simulink model "RTInductionMotorJan27"  (R2019a)
settings: Solver=VariableStepAuto  StartTime=0.0  StopTime=1  RelTol=1e-3
model workspace (MAT data in the model file):
  Fe = 60
  Poles = 2
values from neighbouring files (symbols this model uses):
  Lm = 0.1485    [Setup.m]
  Lr = 0.009061    [Setup.m]
  Ls = 0.003883    [Setup.m]
  Rr = 1.06    [Setup.m]
  Rs = 1    [Setup.m]
libraries: powerlib_meascontrol x1
settings Model: Creator=adam_  LastModifiedBy=adam_

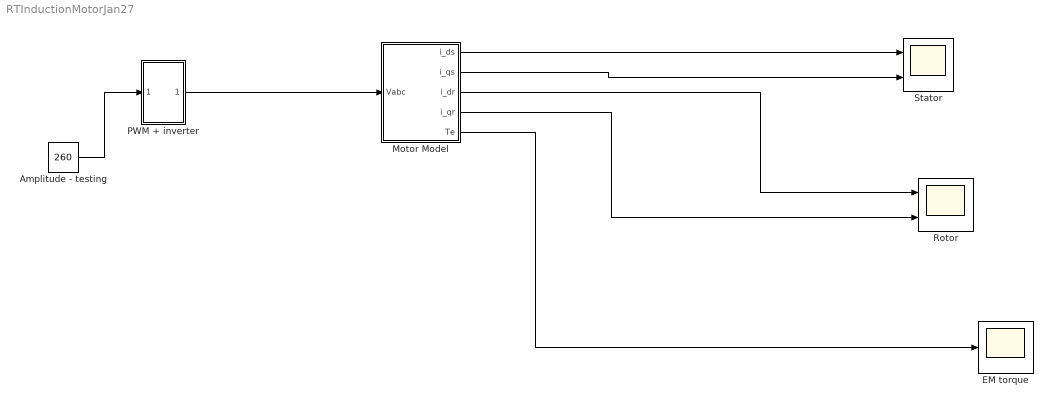
== system RTInductionMotorJan27 ==
  Amplitude - testing : Constant  Value=260
  EM torque : Scope
  Motor Model : Subsystem
  PWM + inverter : Subsystem
  Rotor : Scope  NumInputPorts=2
  Stator : Scope  NumInputPorts=2
  wires:
  PWM + inverter/1(Vabc) -> Motor Model/1(Vabc)
  Motor Model/1(i_ds) -> Stator/1
  Motor Model/2(i_qs) -> Stator/2
  Motor Model/3(i_dr) -> Rotor/1
  Motor Model/4(i_qr) -> Rotor/2
  Motor Model/5(Te) -> EM torque/1
  Amplitude - testing/1 -> PWM + inverter/1(Amplitude)

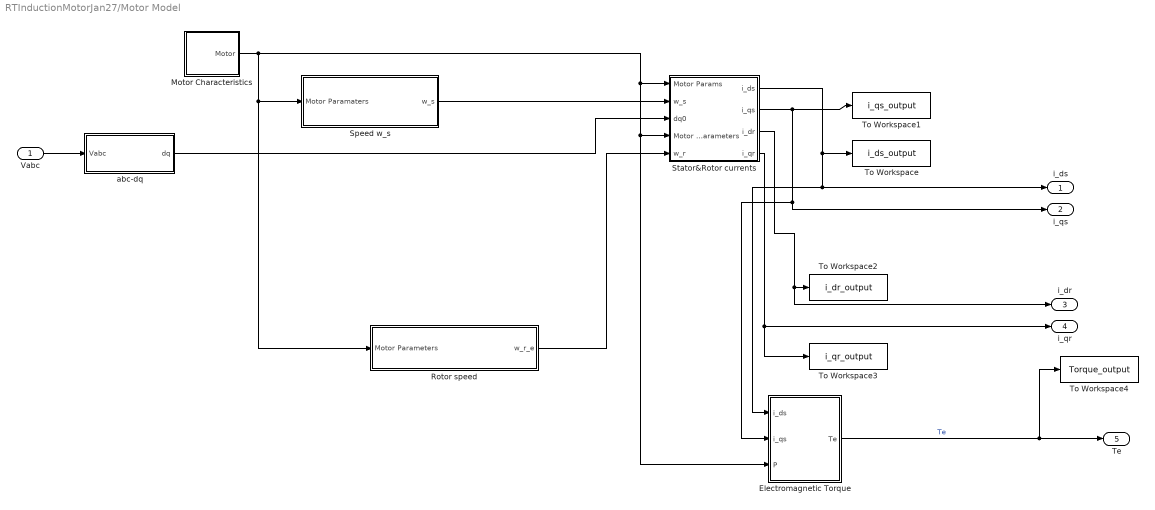
== system RTInductionMotorJan27/Motor Model ==
  Vabc : Inport
  Electromagnetic Torque : Subsystem
  Motor Characteristics : Subsystem
  Rotor speed : Subsystem
  Speed w_s : Subsystem
  Stator&Rotor currents : Subsystem
  To Workspace : ToWorkspace  VariableName=i_ds_output  SaveFormat=Timeseries  SampleTime=-1
  To Workspace1 : ToWorkspace  VariableName=i_qs_output  SaveFormat=Timeseries  SampleTime=-1
  To Workspace2 : ToWorkspace  VariableName=i_dr_output  SaveFormat=Timeseries  SampleTime=-1
  To Workspace3 : ToWorkspace  VariableName=i_qr_output  SaveFormat=Timeseries  SampleTime=-1
  To Workspace4 : ToWorkspace  VariableName=Torque_output  SaveFormat=Timeseries  SampleTime=-1
  abc-dq : Subsystem
  i_ds : Outport
  i_qs : Outport  Port=2
  i_dr : Outport  Port=3
  i_qr : Outport  Port=4
  Te : Outport  Port=5
  wires:
  Vabc/1 -> abc-dq/1(Vabc)
  Rotor speed/1(w_r_e) -> Stator&Rotor currents/5(w_r)
  abc-dq/1(dq) -> Stator&Rotor currents/3(dq0)
  Speed w_s/1(w_s) -> Stator&Rotor currents/2(w_s)
  Stator&Rotor currents/1(i_ds) -> i_ds/1, Electromagnetic Torque/1(i_ds), To Workspace/1
  Motor Characteristics/1(Motor) -> Rotor speed/1(Motor Parameters), Speed w_s/1(Motor Paramaters), Electromagnetic Torque/3(P), Stator&Rotor currents/4(Motor Parameters), Stator&Rotor currents/1(Motor Params)
  Stator&Rotor currents/2(i_qs) -> i_qs/1, Electromagnetic Torque/2(i_qs), To Workspace1/1
  Stator&Rotor currents/4(i_qr) -> i_qr/1, To Workspace3/1
  Stator&Rotor currents/3(i_dr) -> i_dr/1, To Workspace2/1
  Electromagnetic Torque/1(Te) -> Te/1, To Workspace4/1  "Te"

== system RTInductionMotorJan27/PWM + inverter ==
  Amplitude : Inport
  Mux : Mux  Inputs=3
  Product : Product
  Product1 : Product
  Product2 : Product
  Scope : Scope
  Sine Wave : Sin  Frequency=2*pi*60  SampleTime=0
  Sine Wave1 : Sin  Frequency=2*pi*60  Phase=2*pi/3  SampleTime=0
  Sine Wave2 : Sin  Frequency=2*pi*60  Phase=4*pi/3  SampleTime=0
  Three-phase PWM : Subsystem
  Vdc : Constant  Value=360
  inverter : Subsystem
  Vabc : Outport
  wires:
  Mux/1 -> Three-phase PWM/1(Signals)
  Three-phase PWM/1(Pulses) -> inverter/2(Pulses)
  inverter/1(Vabc) -> Vabc/1, Scope/1
  Vdc/1 -> inverter/1(Vdc)
  Sine Wave/1 -> Product/2
  Amplitude/1 -> Product2/1, Product1/1, Product/1
  Product/1 -> Mux/1
  Product2/1 -> Mux/3
  Product1/1 -> Mux/2
  Sine Wave1/1 -> Product1/2
  Sine Wave2/1 -> Product2/2

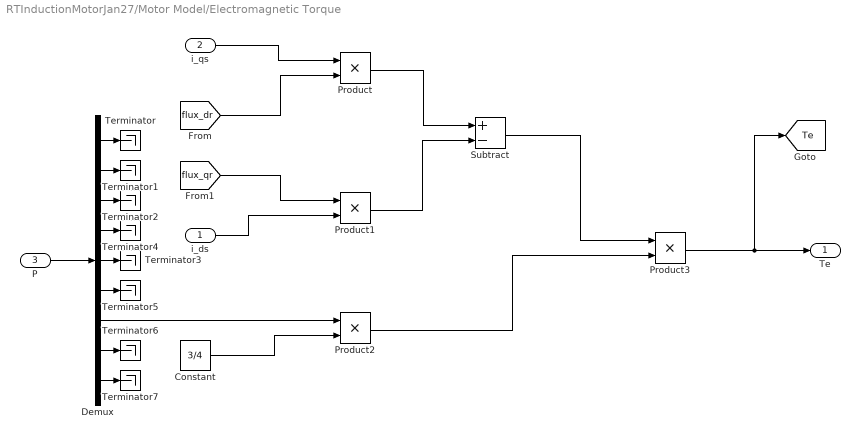
== system RTInductionMotorJan27/Motor Model/Electromagnetic Torque ==
  i_ds : Inport
  i_qs : Inport  Port=2
  P : Inport  Port=3
  Constant : Constant  Value=3/4
  Demux : Demux  Outputs=9
  Product{,1..3} (4 alike) : Product
  Subtract : Sum  Inputs=+-
  Terminator{,1..7} (8 alike) : Terminator
  Te : Outport  VectorParamsAs1DForOutWhenUnconnected=off
  tag scope: Te=global
  wires:
  Product3/1 -> Te/1, [Te]
  Subtract/1 -> Product3/1
  Product2/1 -> Product3/2
  Constant/1 -> Product2/2
  Product1/1 -> Subtract/2
  Product/1 -> Subtract/1
  i_ds/1 -> Product1/2
  [flux_qr] -> Product1/1
  [flux_dr] -> Product/2
  i_qs/1 -> Product/1
  P/1 -> Demux/1
  Demux/7 -> Product2/1
  Demux/1 -> Terminator/1
  Demux/2 -> Terminator1/1
  Demux/3 -> Terminator2/1
  Demux/5 -> Terminator3/1
  Demux/4 -> Terminator4/1
  Demux/6 -> Terminator5/1
  Demux/8 -> Terminator6/1
  Demux/9 -> Terminator7/1

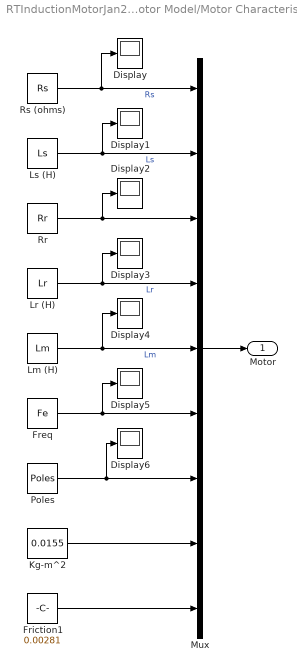
== system RTInductionMotorJan27/Motor Model/Motor Characteristics ==
  Display{,1..6} (7 alike) : Display
  Freq : Constant  Value=Fe
  Friction1 : Constant  Value=0.00281
  Kg-m^2 : Constant  Value=0.0155
  Lm (H) : Constant  Value=Lm
  Lr (H) : Constant  Value=Lr
  Ls (H) : Constant  Value=Ls
  Mux : Mux  Inputs=9
  Poles : Constant  Value=Poles
  Rr : Constant  Value=Rr
  Rs (ohms) : Constant  Value=Rs
  Motor : Outport
  wires:
  Rs (ohms)/1 -> Display/1, Mux/1  "Rs"
  Ls (H)/1 -> Display1/1, Mux/2  "Ls"
  Mux/1 -> Motor/1
  Rr/1 -> Display2/1, Mux/3
  Lr (H)/1 -> Display3/1, Mux/4  "Lr"
  Lm (H)/1 -> Display4/1, Mux/5  "Lm"
  Freq/1 -> Display5/1, Mux/6
  Poles/1 -> Display6/1, Mux/7
  Kg-m^2/1 -> Mux/8
  Friction1/1 -> Mux/9

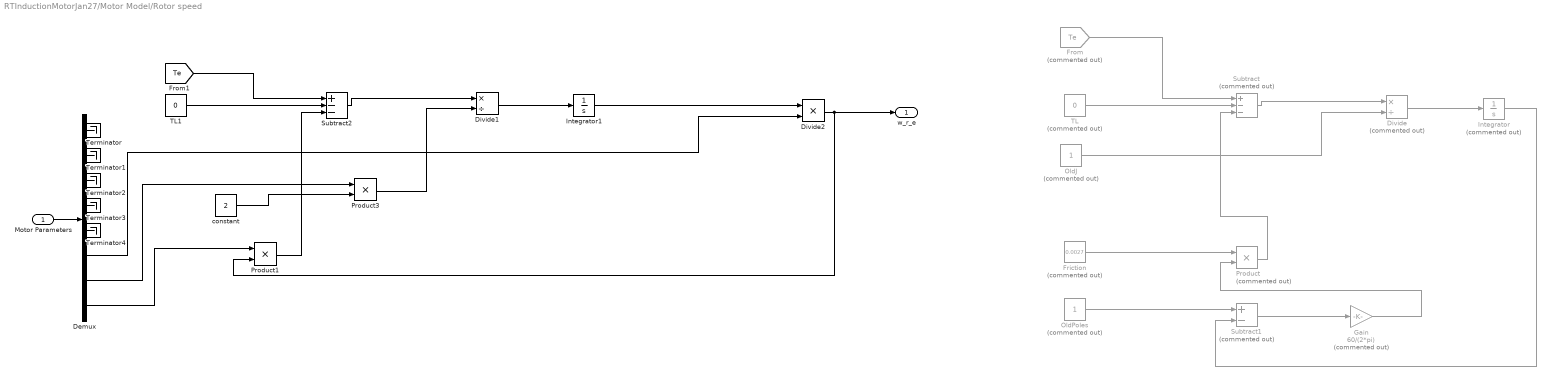
== system RTInductionMotorJan27/Motor Model/Rotor speed ==
  Motor Parameters : Inport
  Demux : Demux  Outputs=8
  Divide : Product  Commented=on  Inputs=*/
  Divide1 : Product  Inputs=*/
  Divide2 : Product  Inputs=**
  Friction : Constant  Commented=on  Value=0.0027
  From : From  Commented=on  GotoTag=Te  TagVisibility=global
  Gain : Gain  Commented=on  Gain=60/(2*pi)
  Integrator : Integrator  Commented=on
  Integrator1 : Integrator
  OldJ : Constant  Commented=on
  OldPoles : Constant  Commented=on
  Product : Product  Commented=on
  Product1 : Product
  Product3 : Product
  Subtract : Sum  Commented=on  Inputs=+--
  Subtract1 : Sum  Commented=on  Inputs=+-
  Subtract2 : Sum  Inputs=+--
  TL : Constant  Commented=on  Value=0
  TL1 : Constant  Value=0
  Terminator{,1..4} (5 alike) : Terminator
  constant : Constant  Value=2
  w_r_e : Outport  VectorParamsAs1DForOutWhenUnconnected=off
  wires:
  From/1 -> Subtract/1
  TL/1 -> Subtract/2
  Subtract/1 -> Divide/1
  Divide/1 -> Integrator/1
  Integrator/1 -> Subtract1/2
  Subtract1/1 -> Gain/1
  Gain/1 -> Product/2
  Friction/1 -> Product/1
  Product/1 -> Subtract/3
  [Te] -> Subtract2/1
  Subtract2/1 -> Divide1/1
  Divide1/1 -> Integrator1/1
  TL1/1 -> Subtract2/2
  Product1/1 -> Subtract2/3
  constant/1 -> Product3/2
  Product3/1 -> Divide1/2
  Integrator1/1 -> Divide2/1
  Demux/6 -> Divide2/2
  Divide2/1 -> Product1/2, w_r_e/1
  Motor Parameters/1 -> Demux/1
  Demux/7 -> Product3/1
  Demux/8 -> Product1/1
  OldJ/1 -> Divide/2
  OldPoles/1 -> Subtract1/1

== system RTInductionMotorJan27/Motor Model/Speed w_s ==
  Motor Paramaters : Inport
  Demux : Demux  Outputs=9
  Divide2 : Product  Inputs=**/
  Terminator{,1..5,7} (7 alike) : Terminator
  constant1 : Constant  Value=120
  rpm to rad/s : Gain  Gain=2*pi/60
  w_s : Outport  VectorParamsAs1DForOutWhenUnconnected=off
  wires:
  constant1/1 -> Divide2/1
  Divide2/1 -> rpm to rad/s/1  "n_s"
  rpm to rad/s/1 -> w_s/1
  Motor Paramaters/1 -> Demux/1
  Demux/6 -> Divide2/2
  Demux/7 -> Divide2/3
  Demux/8 -> Terminator5/1

== system RTInductionMotorJan27/Motor Model/Stator&Rotor currents ==
  Motor Params : Inport
  w_s : Inport  Port=2
  dq0 : Inport  Port=3
  Motor Parameters : Inport  Port=4
  w_r : Inport  Port=5
  Rotor current : Subsystem
  Stator current : Subsystem
  i_ds : Outport
  i_qs : Outport  Port=2
  i_dr : Outport  Port=3
  i_qr : Outport  Port=4
  wires:
  w_s/1 -> Rotor current/2(w_s), Stator current/2(w_s)
  dq0/1 -> Stator current/3(dq0)
  w_r/1 -> Rotor current/3(w_r)
  Stator current/2(i_qs) -> i_qs/1
  Rotor current/1(i_dr) -> i_dr/1
  Motor Parameters/1 -> Rotor current/1(Motor Parameters)
  Motor Params/1 -> Stator current/1(Motor Params)
  Stator current/1(i_ds) -> i_ds/1
  Rotor current/2(i_qr) -> i_qr/1

== system RTInductionMotorJan27/Motor Model/abc-dq ==
  Vabc : Inport
  Add : Sum
  Constant : Constant  Value=2*pi*60
  Constant1 : Constant  Value=-pi/3
  Integrator : Integrator
  Mux3 : Mux  Inputs=2
  Mux4 : Mux  Inputs=2
  Scope2 : Scope
  Scope3 : Scope
  Vd : Fcn  Expr=sqrt(2/3)*(u(1)*cos(u(4))+u(2)*cos(u(4)-2*pi/3)+u(3)*cos(u(4)+2*pi/3))
  Vq : Fcn  Expr=-sqrt(2/3)*(u(1)*sin(u(4))+u(2)*sin(u(4)-2*pi/3)+u(3)*sin(u(4)+2*pi/3))
  dq : Outport  VectorParamsAs1DForOutWhenUnconnected=off
  wires:
  Vabc/1 -> Mux3/1
  Mux3/1 -> Vd/1, Vq/1, Scope2/1
  Constant/1 -> Integrator/1
  Integrator/1 -> Add/1  "w_t"
  Constant1/1 -> Add/2
  Vd/1 -> Mux4/1
  Vq/1 -> Mux4/2
  Mux4/1 -> dq/1, Scope3/1
  Add/1 -> Mux3/2

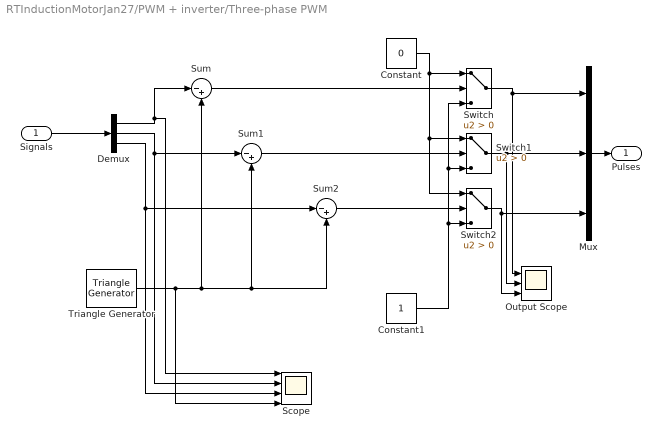
== system RTInductionMotorJan27/PWM + inverter/Three-phase PWM ==
  Signals : Inport
  Constant : Constant  Value=0
  Constant1 : Constant
  Demux : Demux  Outputs=3
  Mux : Mux  Inputs=3
  Output Scope : Scope  NumInputPorts=3
  Scope : Scope  NumInputPorts=4
  Sum : Sum  Inputs=|-+
  Sum1 : Sum  Inputs=|-+
  Sum2 : Sum  Inputs=|-+
  Switch : Switch  Criteria=u2 > Threshold
  Switch1 : Switch  Criteria=u2 > Threshold
  Switch2 : Switch  Criteria=u2 > Threshold
  Triangle Generator : powerlib_meascontrol/Pulse & Signal Generators/Triangle Generator  Freq=fs  Phase=90  Ts=1e-6
  Pulses : Outport
  wires:
  Sum/1 -> Switch/2
  Triangle Generator/1 -> Scope/4, Sum2/2, Sum1/2, Sum/2
  Constant/1 -> Switch2/1, Switch1/1, Switch/1
  Switch1/1 -> Output Scope/2, Mux/2
  Demux/2 -> Scope/2, Sum1/1
  Switch2/1 -> Output Scope/3, Mux/3
  Constant1/1 -> Switch1/3, Switch/3, Switch2/3
  Switch/1 -> Output Scope/1, Mux/1
  Demux/3 -> Scope/3, Sum2/1
  Sum1/1 -> Switch1/2
  Sum2/1 -> Switch2/2
  Mux/1 -> Pulses/1
  Signals/1 -> Demux/1
  Demux/1 -> Scope/1, Sum/1

== system RTInductionMotorJan27/PWM + inverter/inverter ==
  Vdc : Inport
  Pulses : Inport  Port=2
  Mux : Mux  Inputs=2
  Mux1 : Mux  Inputs=3
  Scope : Scope  NumInputPorts=3
  vaN : Fcn  Expr=u(1)*((2*u(2))-u(3)-u(4))/3
  vbN : Fcn  Expr=u(1)*((2*u(3))-u(2)-u(4))/3
  vcN : Fcn  Expr=u(1)*((2*u(4))-u(3)-u(2))/3
  Vabc : Outport
  wires:
  Vdc/1 -> Mux/1
  Pulses/1 -> Mux/2
  Mux/1 -> vcN/1, vbN/1, vaN/1
  Mux1/1 -> Vabc/1
  vaN/1 -> Scope/1, Mux1/1
  vbN/1 -> Scope/2, Mux1/2
  vcN/1 -> Mux1/3, Scope/3

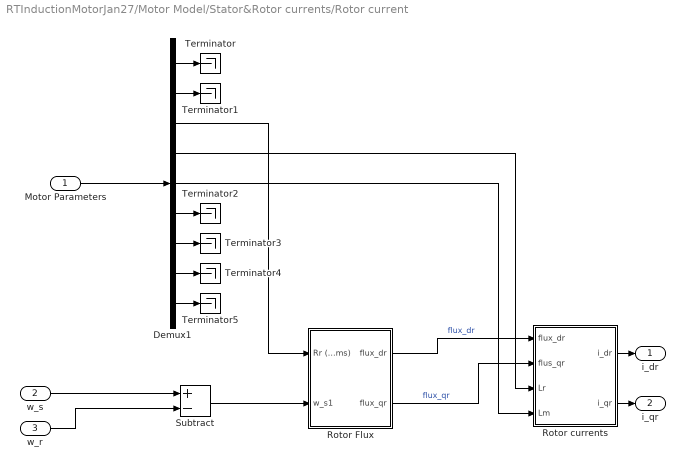
== system RTInductionMotorJan27/Motor Model/Stator&Rotor currents/Rotor current ==
  Motor Parameters : Inport
  w_s : Inport  Port=2
  w_r : Inport  Port=3
  Demux1 : Demux  Outputs=9
  Rotor Flux : Subsystem
  Rotor currents : Subsystem
  Subtract : Sum  Inputs=+-
  Terminator{,1..5} (6 alike) : Terminator
  i_dr : Outport  VectorParamsAs1DForOutWhenUnconnected=off
  i_qr : Outport  Port=2  VectorParamsAs1DForOutWhenUnconnected=off
  wires:
  Subtract/1 -> Rotor Flux/2(w_s1)
  w_r/1 -> Subtract/2
  Rotor currents/2(i_qr) -> i_qr/1
  Rotor currents/1(i_dr) -> i_dr/1
  Rotor Flux/1(flux_dr) -> Rotor currents/1(flux_dr)  "flux_dr"
  Rotor Flux/2(flux_qr) -> Rotor currents/2(flus_qr)  "flux_qr"
  w_s/1 -> Subtract/1
  Motor Parameters/1 -> Demux1/1
  Demux1/3 -> Rotor Flux/1(Rr (Ohms))
  Demux1/4 -> Rotor currents/3(Lr)
  Demux1/5 -> Rotor currents/4(Lm)
  Demux1/1 -> Terminator/1
  Demux1/2 -> Terminator1/1
  Demux1/6 -> Terminator2/1
  Demux1/7 -> Terminator3/1
  Demux1/8 -> Terminator4/1
  Demux1/9 -> Terminator5/1

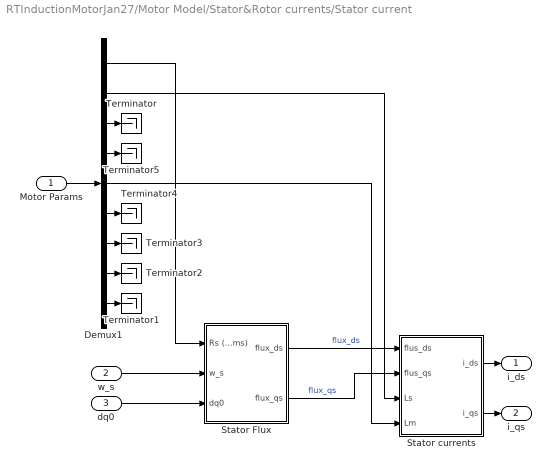
== system RTInductionMotorJan27/Motor Model/Stator&Rotor currents/Stator current ==
  Motor Params : Inport
  w_s : Inport  Port=2
  dq0 : Inport  Port=3
  Demux1 : Demux  Outputs=9
  Stator Flux : Subsystem
  Stator currents : Subsystem
  Terminator{,1..5} (6 alike) : Terminator
  i_ds : Outport  VectorParamsAs1DForOutWhenUnconnected=off
  i_qs : Outport  Port=2  VectorParamsAs1DForOutWhenUnconnected=off
  wires:
  dq0/1 -> Stator Flux/3(dq0)
  Stator currents/2(i_qs) -> i_qs/1
  w_s/1 -> Stator Flux/2(w_s)
  Stator currents/1(i_ds) -> i_ds/1
  Stator Flux/1(flux_ds) -> Stator currents/1(flus_ds)  "flux_ds"
  Stator Flux/2(flux_qs) -> Stator currents/2(flus_qs)  "flux_qs"
  Motor Params/1 -> Demux1/1
  Demux1/1 -> Stator Flux/1(Rs (Ohms))
  Demux1/2 -> Stator currents/3(Ls)
  Demux1/5 -> Stator currents/4(Lm)
  Demux1/3 -> Terminator/1
  Demux1/4 -> Terminator5/1
  Demux1/6 -> Terminator4/1
  Demux1/7 -> Terminator3/1
  Demux1/8 -> Terminator2/1
  Demux1/9 -> Terminator1/1

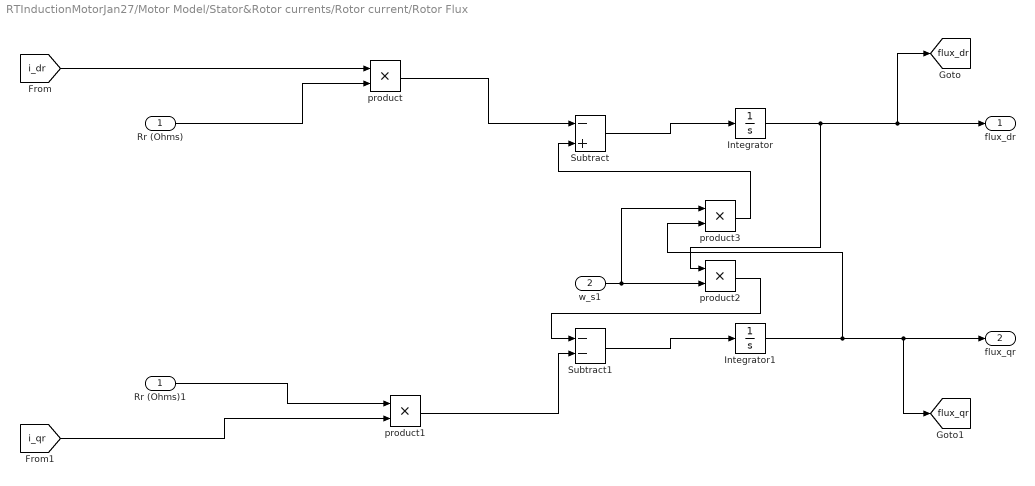
== system RTInductionMotorJan27/Motor Model/Stator&Rotor currents/Rotor current/Rotor Flux ==
  Rr (Ohms) : Inport
  w_s1 : Inport  Port=2
  Integrator : Integrator
  Integrator1 : Integrator
  Rr (Ohms)1 : InportShadow
  Subtract : Sum  Inputs=-+
  Subtract1 : Sum  Inputs=--
  product{,1..3} (4 alike) : Product  Inputs=**
  flux_dr : Outport  VectorParamsAs1DForOutWhenUnconnected=off
  flux_qr : Outport  Port=2  VectorParamsAs1DForOutWhenUnconnected=off
  tag scope: flux_dr=global, flux_qr=global
  wires:
  [i_qr] -> product1/2
  product2/1 -> Subtract1/1
  product3/1 -> Subtract/2
  w_s1/1 -> product2/2, product3/1
  Rr (Ohms)1/1 -> product1/1
  Integrator1/1 -> flux_qr/1, [flux_qr], product3/2
  [i_dr] -> product/1
  product1/1 -> Subtract1/2
  Subtract1/1 -> Integrator1/1
  Integrator/1 -> flux_dr/1, [flux_dr], product2/1
  Subtract/1 -> Integrator/1
  product/1 -> Subtract/1
  Rr (Ohms)/1 -> product/2

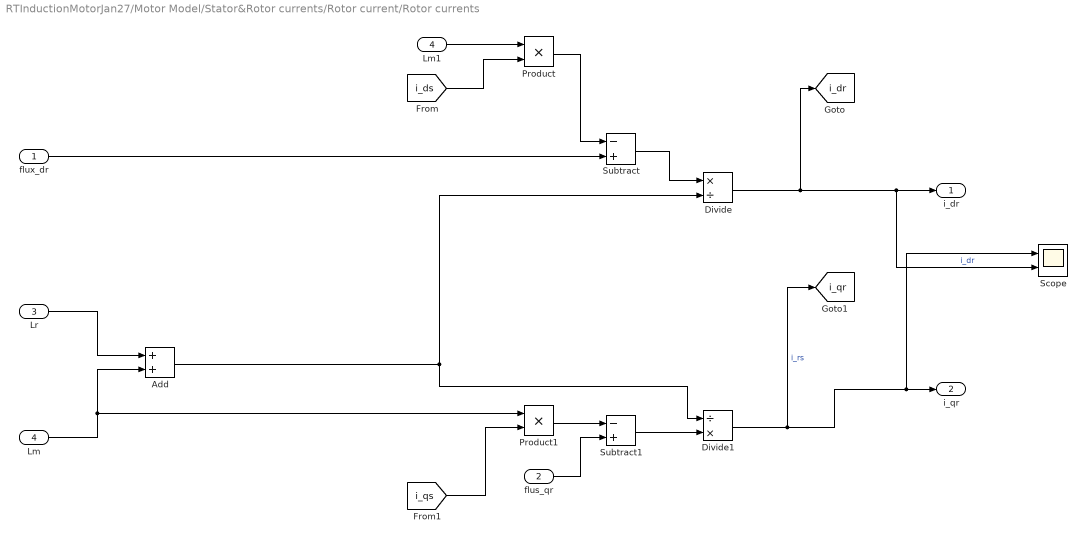
== system RTInductionMotorJan27/Motor Model/Stator&Rotor currents/Rotor current/Rotor currents ==
  flux_dr : Inport
  flus_qr : Inport  Port=2
  Lr : Inport  Port=3
  Lm : Inport  Port=4
  Add : Sum
  Divide : Product  Inputs=*/
  Divide1 : Product  Inputs=/*
  Lm1 : InportShadow  Port=4
  Product : Product
  Product1 : Product
  Scope : Scope  NumInputPorts=2
  Subtract : Sum  Inputs=-+
  Subtract1 : Sum  Inputs=-+
  i_dr : Outport  VectorParamsAs1DForOutWhenUnconnected=off
  i_qr : Outport  Port=2  VectorParamsAs1DForOutWhenUnconnected=off
  tag scope: i_dr=global, i_qr=global
  wires:
  Divide1/1 -> i_qr/1, Scope/1, [i_qr]  "i_rs"
  Subtract1/1 -> Divide1/2
  flus_qr/1 -> Subtract1/2
  Product1/1 -> Subtract1/1
  [i_qs] -> Product1/2
  Divide/1 -> i_dr/1, Scope/2, [i_dr]  "i_dr"
  Add/1 -> Divide/2, Divide1/1
  Subtract/1 -> Divide/1
  Lm/1 -> Add/2, Product1/1
  Lr/1 -> Add/1
  Product/1 -> Subtract/1
  flux_dr/1 -> Subtract/2
  [i_ds] -> Product/2
  Lm1/1 -> Product/1

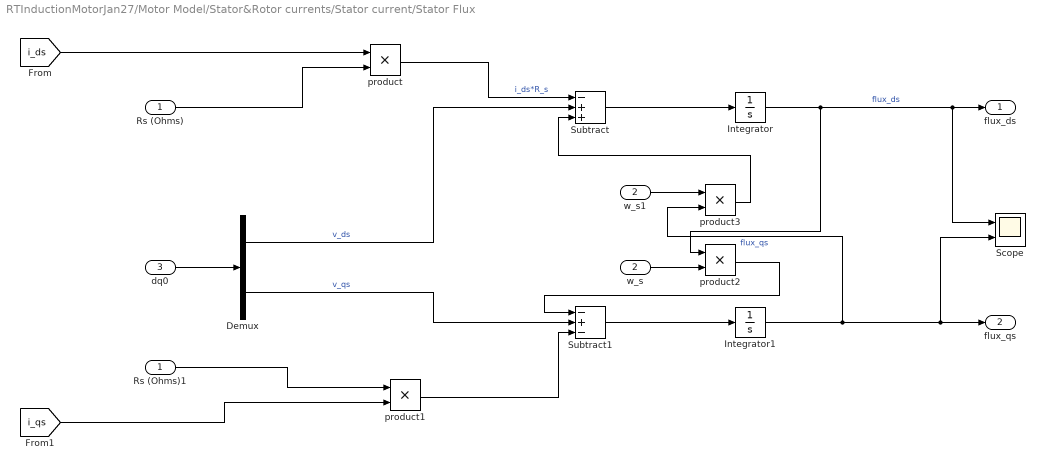
== system RTInductionMotorJan27/Motor Model/Stator&Rotor currents/Stator current/Stator Flux ==
  Rs (Ohms) : Inport
  w_s : Inport  Port=2
  dq0 : Inport  Port=3
  Demux : Demux  Outputs=2
  Integrator : Integrator
  Integrator1 : Integrator
  Rs (Ohms)1 : InportShadow
  Scope : Scope  NumInputPorts=2
  Subtract : Sum  Inputs=-++
  Subtract1 : Sum  Inputs=-+-
  product{,1..3} (4 alike) : Product  Inputs=**
  w_s1 : InportShadow  Port=2
  flux_ds : Outport  VectorParamsAs1DForOutWhenUnconnected=off
  flux_qs : Outport  Port=2  VectorParamsAs1DForOutWhenUnconnected=off
  wires:
  Demux/2 -> Subtract1/2  "v_qs"
  Demux/1 -> Subtract/2  "v_ds"
  [i_qs] -> product1/2
  product2/1 -> Subtract1/1
  w_s/1 -> product2/2
  product3/1 -> Subtract/3
  w_s1/1 -> product3/1
  Rs (Ohms)1/1 -> product1/1
  Integrator1/1 -> flux_qs/1, Scope/2, product3/2  "flux_qs"
  [i_ds] -> product/1
  product1/1 -> Subtract1/3
  Subtract1/1 -> Integrator1/1
  Integrator/1 -> flux_ds/1, Scope/1, product2/1  "flux_ds"
  Subtract/1 -> Integrator/1
  product/1 -> Subtract/1  "i_ds*R_s"
  Rs (Ohms)/1 -> product/2
  dq0/1 -> Demux/1

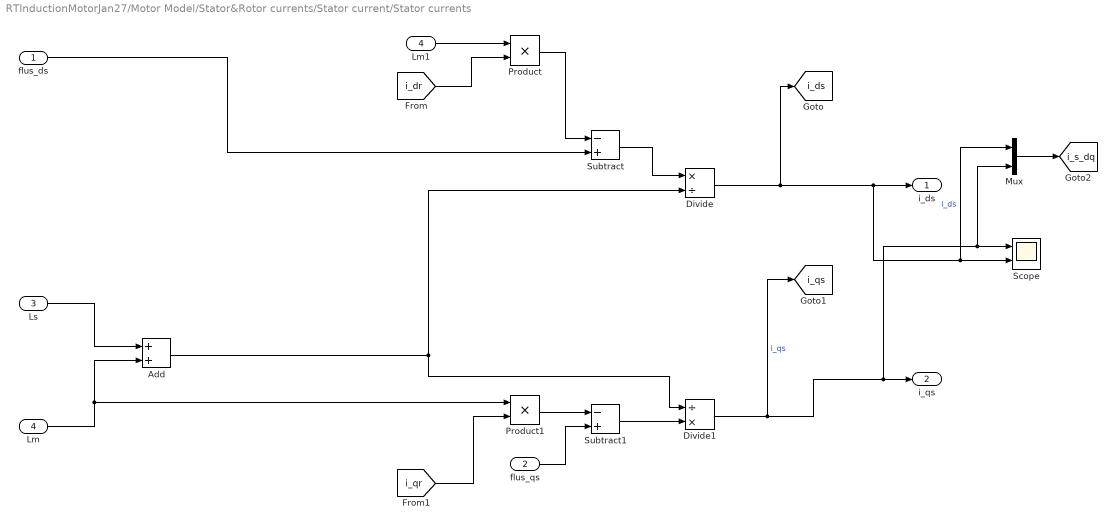
== system RTInductionMotorJan27/Motor Model/Stator&Rotor currents/Stator current/Stator currents ==
  flus_ds : Inport
  flus_qs : Inport  Port=2
  Ls : Inport  Port=3
  Lm : Inport  Port=4
  Add : Sum
  Divide : Product  Inputs=*/
  Divide1 : Product  Inputs=/*
  Lm1 : InportShadow  Port=4
  Mux : Mux  Inputs=2
  Product : Product
  Product1 : Product
  Scope : Scope  NumInputPorts=2
  Subtract : Sum  Inputs=-+
  Subtract1 : Sum  Inputs=-+
  i_ds : Outport  VectorParamsAs1DForOutWhenUnconnected=off
  i_qs : Outport  Port=2  VectorParamsAs1DForOutWhenUnconnected=off
  tag scope: i_ds=global, i_qs=global, i_s_dq=global
  wires:
  Mux/1 -> [i_s_dq]
  Divide1/1 -> i_qs/1, Scope/1, Mux/2, [i_qs]  "i_qs"
  Subtract1/1 -> Divide1/2
  flus_qs/1 -> Subtract1/2
  Product1/1 -> Subtract1/1
  [i_qr] -> Product1/2
  Divide/1 -> i_ds/1, Scope/2, Mux/1, [i_ds]  "i_ds"
  Add/1 -> Divide/2, Divide1/1
  Subtract/1 -> Divide/1
  Lm/1 -> Add/2, Product1/1
  Ls/1 -> Add/1
  Product/1 -> Subtract/1
  flus_ds/1 -> Subtract/2
  [i_dr] -> Product/2
  Lm1/1 -> Product/1
